simulink model "Active_Suspension_model"  (R2022b)
settings: Solver=ode1  StartTime=0.0  StopTime=10  FixedStep=0.001  MaxStep=0.1  RelTol=1e-3
values from neighbouring files (symbols this model uses):
  A = [   0       1        0          -1 ... (first row only)    [main.m]    (also in quarter_car_main.m)
  B = [  0       0 ... (first row only)    [main.m]    (also in quarter_car_main.m)
  C = [        eye(4) ... (first row only)    [main.m]    (also in quarter_car_main.m)
  D = [zeros(4,2) ... (first row only)    [main.m]    (also in quarter_car_main.m)
  K = lqr( A, B(:,2), Q, R )    [main.m]    (also in quarter_car_main.m)
libraries: slpidlib x1
settings Model: Creator=giacomo  LastModifiedBy=giacomo

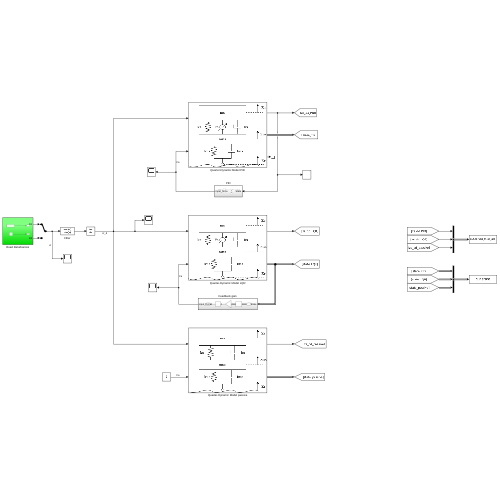
[thumbnail: Simulink's stored preview of the top-level diagram]
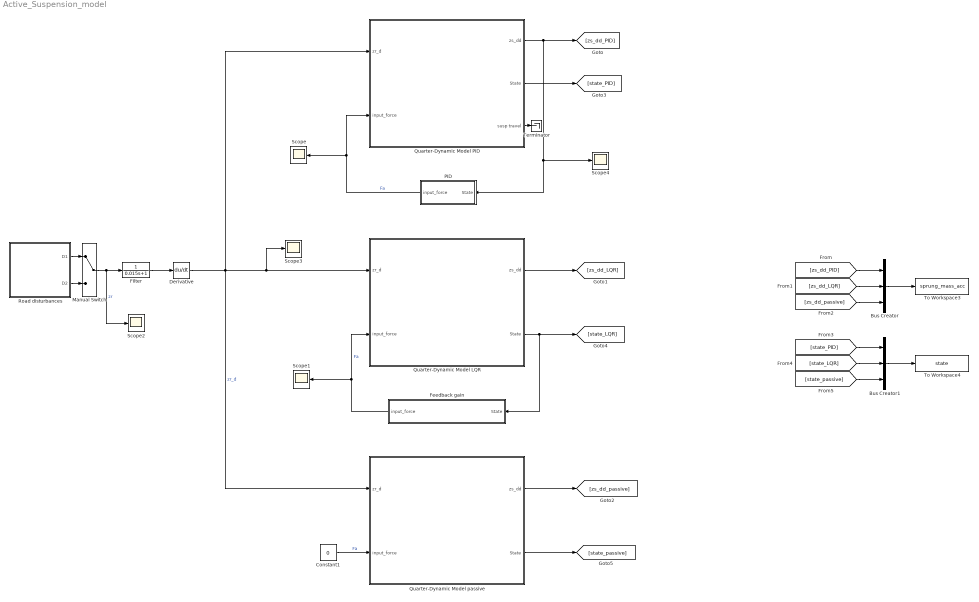
== system Active_Suspension_model ==
  Bus Creator : BusCreator  Inputs=3
  Bus Creator1 : BusCreator  Inputs=3
  Constant1 : Constant  Value=0
  Derivative : Derivative
  FIlter : TransferFcn  Denominator=[0.015 1]
  Feedback gain : Subsystem
  Manual Switch : ManualSwitch
  PID : Subsystem
  Quarter-Dynamic Model LQR : Subsystem
      mask Display: image('/home/giacomo/University/Active_suspension/imgs/Active_susp.png'); % Use "Edit Image" on toolstrip to change.
  Quarter-Dynamic Model PID : Subsystem
      mask Display: image('/home/giacomo/University/Active_suspension/imgs/Active_susp.png'); % Use "Edit Image" on toolstrip to change.
  Quarter-Dynamic Model passive : Subsystem
      mask Display: image('/home/giacomo/University/Active_suspension/imgs/Passive_susp.png'); % Use "Edit Image" on toolstrip to change.
  Road disturbances : Subsystem
  Scope{,1..4} (5 alike) : Scope
  Terminator : Terminator
  To Workspace3 : ToWorkspace  VariableName=sprung_mass_acc  SaveFormat=Timeseries  SampleTime=-1
  To Workspace4 : ToWorkspace  VariableName=state  SaveFormat=Timeseries  SampleTime=-1
  wires:
  Road disturbances/1(D1) -> Manual Switch/1
  Road disturbances/2(D2) -> Manual Switch/2
  Manual Switch/1 -> Scope2/1, FIlter/1  "zr"
  Constant1/1 -> Quarter-Dynamic Model passive/2(input_force)  "Fa"
  Derivative/1 -> Scope3/1, Quarter-Dynamic Model LQR/1(zr_d), Quarter-Dynamic Model PID/1(zr_d), Quarter-Dynamic Model passive/1(zr_d)  "zr_d"
  Feedback gain/1(input_force) -> Scope1/1, Quarter-Dynamic Model LQR/2(input_force)  "Fa"
  PID/1(input_force) -> Quarter-Dynamic Model PID/2(input_force), Scope/1  "Fa"
  Quarter-Dynamic Model PID/1(zs_dd) -> [zs_dd_PID], Scope4/1, PID/1(State)
  Quarter-Dynamic Model passive/2(State) -> [state_passive]
  Quarter-Dynamic Model LQR/2(State) -> [state_LQR], Feedback gain/1(State)
  Quarter-Dynamic Model PID/2(State) -> [state_PID]
  Quarter-Dynamic Model LQR/1(zs_dd) -> [zs_dd_LQR]
  Quarter-Dynamic Model passive/1(zs_dd) -> [zs_dd_passive]
  [zs_dd_PID] -> Bus Creator/1
  [zs_dd_passive] -> Bus Creator/3
  [zs_dd_LQR] -> Bus Creator/2
  Bus Creator/1 -> To Workspace3/1
  [state_PID] -> Bus Creator1/1
  [state_LQR] -> Bus Creator1/2
  [state_passive] -> Bus Creator1/3
  Bus Creator1/1 -> To Workspace4/1
  FIlter/1 -> Derivative/1
  Quarter-Dynamic Model PID/3(susp travel) -> Terminator/1

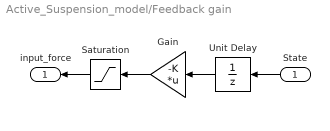
== system Active_Suspension_model/Feedback gain ==
  State : Inport
  Gain : Gain  Gain=-K  Multiplication=Matrix(K*u)
  Saturation : Saturate  UpperLimit=46730  LowerLimit=-46730
  Unit Delay : UnitDelay  SampleTime=-1  HasFrameUpgradeWarning=on
  input_force : Outport
  wires:
  Unit Delay/1 -> Gain/1
  Gain/1 -> Saturation/1
  Saturation/1 -> input_force/1
  State/1 -> Unit Delay/1

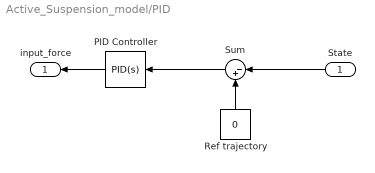
== system Active_Suspension_model/PID ==
  State : Inport
  PID Controller : slpidlib/PID Controller  Controller=PID  Form=Parallel  TimeDomain=Continuous-time  UseExternalTs=off  SampleTime=-1  IntegratorMethod=Forward Euler  FilterMethod=Forward Euler  ControllerParametersSource=internal  P=1000  I=50  UseKiTs=off  D=150  N=100  UseFilter=on  TunerSelectOption=Transfer Function Based (PID Tuner App)  InitialConditionSource=internal  InitialConditionForIntegrator=0  InitialConditionForFilter=0  DifferentiatorICPrevScaledInput=0  ExternalReset=none  TrackingMode=off  Kt=1  LimitOutput=off  SatLimitsSource=internal  UpperSaturationLimit=inf  LowerSaturationLimit=-inf  LinearizeAsGain=on  AntiWindupMode=none  Kb=1  LimitIntegrator=off  UpperIntegratorSaturationLimit=inf  LowerIntegratorSaturationLimit=-inf  POutMin=[]  POutMax=[]  IOutMin=[]  IOutMax=[]  DOutMin=[]  DOutMax=[]  NOutMin=[]  NOutMax=[]  SumOutMin=[]  SumOutMax=[]  SaturationOutMin=[]  SaturationOutMax=[]  PParamMin=[]  PParamMax=[]  IParamMin=[]  IParamMax=[]  DParamMin=[]  DParamMax=[]  NParamMin=[]  NParamMax=[]  KbParamMin=[]  KbParamMax=[]  KtParamMin=[]  KtParamMax=[]  KbOutMin=[]  KbOutMax=[]  KtOutMin=[]  KtOutMax=[]  IntegratorOutMin=[]  IntegratorOutMax=[]  FilterOutMin=[]  FilterOutMax=[]  SumI1OutMin=[]  SumI1OutMax=[]  SumI2OutMin=[]  SumI2OutMax=[]  SumI3OutMin=[]  SumI3OutMax=[]  SumI4OutMin=[]  SumI4OutMax=[]  SumDOutMin=[]  SumDOutMax=[]  DifferentiatorOutMin=[]  DifferentiatorOutMax=[]  FilterDiffOutCoefMin=[]  FilterDiffOutCoefMax=[]  ReciprocalOutMin=[]  ReciprocalOutMax=[]  SumDenOutMin=[]  SumDenOutMax=[]  SumNumOutMin=[]  SumNumOutMax=[]  DivideOutMin=[]  DivideOutMax=[]  UdiffTsProdOutMin=[]  UdiffTsProdOutMax=[]  NTsProdOutMin=[]  NTsProdOutMax=[]  UintegralTsProdOutMin=[]  UintegralTsProdOutMax=[]  UngainTsProdOutMin=[]  UngainTsProdOutMax=[]  ClampingZeroOutDataTypeStr=Inherit: Inherit via back propagation  ClampingZeroOutMin=[]  ClampingZeroOutMax=[]  FilterDenConstantOutDataTypeStr=Inherit: Inherit via back propagation  FilterDenConstantOutMin=[]  FilterDenConstantOutMax=[]  PCopyOutDataTypeStr=Inherit: Inherit via back propagation  PCopyOutMin=[]  PCopyOutMax=[]  NCopyOutDataTypeStr=Inherit: Inherit via back propagation  NCopyOutMin=[]  NCopyOutMax=[]  IntegratorContinuousStateAttributes=''  IntegratorStateMustResolveToSignalObject=off  IntegratorRTWStateStorageClass=Auto  FilterContinuousStateAttributes=''  FilterStateMustResolveToSignalObject=off  FilterRTWStateStorageClass=Auto  ParallelPVariant=InternalParameters  IdealPVariant=Disabled  IVariant=InternalParameters  DVariant=InternalParameters  IntegratorVariant=Continuous  SatVariant=Disabled  AWVariant=Passthrough  PCopyVariant=Disabled  TRVariant=Disabled  FdbkBlocksVariant=Forward  IdealPFdbkVariant=Disabled  SatFdbkVariant=Disabled  DerivativeFilterVariant=ContFilter  NVariant=InternalParameters  NCopyVariant=Disabled  FilterICVariant=InternalICsFilter  IntegratorICVariant=InternalICs  ExternalResetVariant=Disabled  TRSumVariant=Passthrough  SumFdbkVariant=Disabled  SumVariant=Sum_PID  TsampFilterVariant=InternalTs  TsampNgainVariant=Passthrough  TsampIntegralVariant=Passthrough  ExternalSaturationOutDataTypeStr=Inherit: Same as second input
  Ref trajectory : Constant  Value=0
  Sum : Sum  Inputs=|-+
  input_force : Outport
  wires:
  Ref trajectory/1 -> Sum/2
  Sum/1 -> PID Controller/1
  PID Controller/1 -> input_force/1
  State/1 -> Sum/1

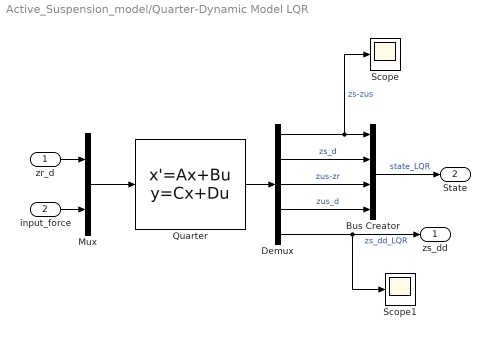
== system Active_Suspension_model/Quarter-Dynamic Model LQR ==
  zr_d : Inport
  input_force : Inport  Port=2
  Bus Creator : BusCreator  Inputs=4
  Demux : Demux  Outputs=5
  Mux : Mux  Inputs=2
  Quarter : StateSpace  A=A  B=B  C=C  D=D  InitialCondition=0
  Scope : Scope
  Scope1 : Scope
  zs_dd : Outport
  State : Outport  Port=2
  wires:
  Mux/1 -> Quarter/1
  zr_d/1 -> Mux/1
  input_force/1 -> Mux/2
  Quarter/1 -> Demux/1
  Demux/1 -> Scope/1, Bus Creator/1  "zs-zus"
  Demux/2 -> Bus Creator/2  "zs_d"
  Demux/3 -> Bus Creator/3  "zus-zr"
  Demux/4 -> Bus Creator/4  "zus_d"
  Bus Creator/1 -> State/1  "state_LQR"
  Demux/5 -> Scope1/1, zs_dd/1  "zs_dd_LQR"

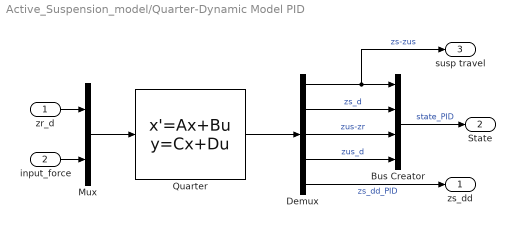
== system Active_Suspension_model/Quarter-Dynamic Model PID ==
  zr_d : Inport
  input_force : Inport  Port=2
  Bus Creator : BusCreator  Inputs=4
  Demux : Demux  Outputs=5
  Mux : Mux  Inputs=2
  Quarter : StateSpace  A=A  B=B  C=C  D=D  InitialCondition=0
  zs_dd : Outport
  State : Outport  Port=2
  susp travel : Outport  Port=3
  wires:
  Mux/1 -> Quarter/1
  zr_d/1 -> Mux/1
  input_force/1 -> Mux/2
  Demux/3 -> Bus Creator/3  "zus-zr"
  Demux/1 -> Bus Creator/1, susp travel/1  "zs-zus"
  Demux/2 -> Bus Creator/2  "zs_d"
  Bus Creator/1 -> State/1  "state_PID"
  Quarter/1 -> Demux/1
  Demux/4 -> Bus Creator/4  "zus_d"
  Demux/5 -> zs_dd/1  "zs_dd_PID"

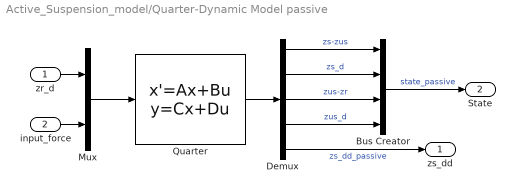
== system Active_Suspension_model/Quarter-Dynamic Model passive ==
  zr_d : Inport
  input_force : Inport  Port=2
  Bus Creator : BusCreator  Inputs=4
  Demux : Demux  Outputs=5
  Mux : Mux  Inputs=2
  Quarter : StateSpace  A=A  B=B  C=C  D=D  InitialCondition=0
  zs_dd : Outport
  State : Outport  Port=2
  wires:
  Mux/1 -> Quarter/1
  zr_d/1 -> Mux/1
  input_force/1 -> Mux/2
  Demux/3 -> Bus Creator/3  "zus-zr"
  Demux/2 -> Bus Creator/2  "zs_d"
  Quarter/1 -> Demux/1
  Bus Creator/1 -> State/1  "state_passive"
  Demux/4 -> Bus Creator/4  "zus_d"
  Demux/1 -> Bus Creator/1  "zs-zus"
  Demux/5 -> zs_dd/1  "zs_dd_passive"

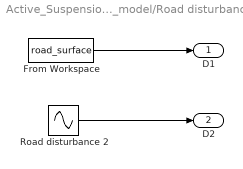
== system Active_Suspension_model/Road disturbances ==
  From Workspace : FromWorkspace  VariableName=road_surface
  Road disturbance 2 : Sin  Frequency=2*pi  SampleTime=0
  D1 : Outport
  D2 : Outport  Port=2
  wires:
  From Workspace/1 -> D1/1
  Road disturbance 2/1 -> D2/1
